simulink model "ballBeam"  (R2017a)
settings: Solver=ode45  StartTime=0.0  StopTime=10.0  RelTol=1e-3
values from neighbouring files (symbols this model uses):
  d = 0.03    [setup_ball_beam.m]
  g = -9.8    [setup_ball_beam.m]
  J = 9.99e-6    (= 9.99e-06)    [setup_ball_beam.m]
  L = 1.0    (= 1)    [setup_ball_beam.m]
  m = 0.111    [setup_ball_beam.m]
  R = 0.015    [setup_ball_beam.m]
settings Model: Creator=sansh  LastModifiedBy=sansh

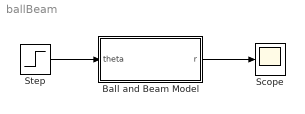
== system ballBeam ==
  Ball and Beam Model : Subsystem
  Scope : Scope
  Step : Step  Time=0  SampleTime=0
  wires:
  Step/1 -> Ball and Beam Model/1(theta)
  Ball and Beam Model/1(r) -> Scope/1

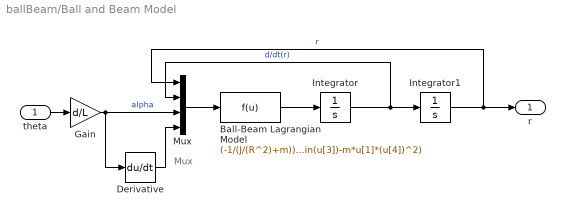
== system ballBeam/Ball and Beam Model ==
  note: Mux
  theta : Inport
  Ball-Beam Lagrangian Model : Fcn  Expr=(-1/(J/(R^2)+m))*(m*g*sin(u[3])-m*u[1]*(u[4])^2)
  Derivative : Derivative
  Gain : Gain  Gain=d/L
  Integrator : Integrator
  Integrator1 : Integrator
  Mux : Mux
  r : Outport
  wires:
  theta/1 -> Gain/1
  Gain/1 -> Derivative/1, Mux/3  "alpha"
  Ball-Beam Lagrangian Model/1 -> Integrator/1
  Derivative/1 -> Mux/4
  Integrator1/1 -> Mux/1, r/1  "r"
  Mux/1 -> Ball-Beam Lagrangian Model/1
  Integrator/1 -> Mux/2, Integrator1/1  "d/dt(r)"
